simulink model "untitled"  (Simulink 7.5)
settings: Solver=ode45  StartTime=0.0  StopTime=1.4  RelTol=1e-3
libraries: fl_lib x38, nesl_utility x3
settings Model: Creator=USUARIO  LastModifiedBy=davito

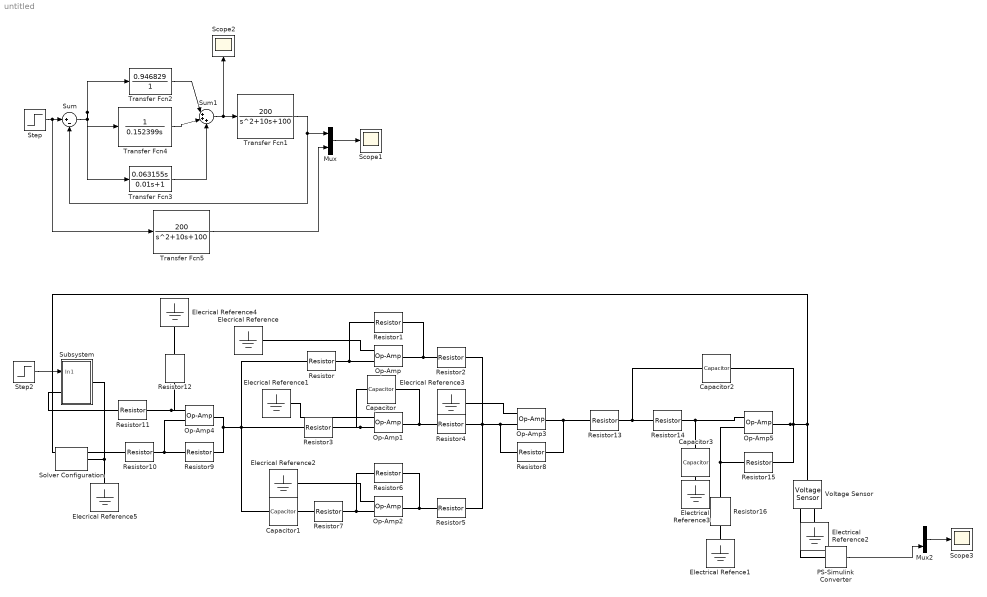
== system untitled ==
  Capacitor : fl_lib/Electrical/Electrical Elements/Capacitor  DialogController=NetworkEngine.DynNeDlgSource  SystemSampleTime=-1  c=10e-6 F  v0=0 V  r=1e-6 Ohm  g=0 1/Ohm  i_Log=off  v_Log=off  vc_Log=off  LocalVarNames=|i|v|vc  LocalVarDescs=|i|v|Internal variable for voltage across capacitor term  LocalVarLogging=[0 0 0]
  Capacitor1 : fl_lib/Electrical/Electrical Elements/Capacitor  DialogController=NetworkEngine.DynNeDlgSource  SystemSampleTime=-1  c=10e-6 F  v0=0 V  r=1e-6 Ohm  g=0 1/Ohm  i_Log=off  v_Log=off  vc_Log=off  LocalVarNames=|i|v|vc  LocalVarDescs=|i|v|Internal variable for voltage across capacitor term  LocalVarLogging=[0 0 0]
  Capacitor2 : fl_lib/Electrical/Electrical Elements/Capacitor  DialogController=NetworkEngine.DynNeDlgSource  SystemSampleTime=-1  c=10.97e-06 F  v0=0 V  r=1e-06 Ohm  g=0 1/Ohm  i_Log=off  v_Log=off  vc_Log=off  LocalVarNames=|i|v|vc  LocalVarDescs=|i|v|Internal variable for voltage across capacitor term  LocalVarLogging=[0 0 0]
  Capacitor3 : fl_lib/Electrical/Electrical Elements/Capacitor  DialogController=NetworkEngine.DynNeDlgSource  SystemSampleTime=-1  c=10.49e-06 F  v0=0 V  r=1e-06 Ohm  g=0 1/Ohm  i_Log=off  v_Log=off  vc_Log=off  LocalVarNames=|i|v|vc  LocalVarDescs=|i|v|Internal variable for voltage across capacitor term  LocalVarLogging=[0 0 0]
  Elecrical Reference{,1..5} (6 alike) : fl_lib/Electrical/Electrical Elements/Electrical Reference  DialogController=NetworkEngine.DynNeDlgSource  SystemSampleTime=-1  i_Log=off  LocalVarNames=|i  LocalVarDescs=|i  LocalVarLogging=0
  Electrical Refence1 : fl_lib/Electrical/Electrical Elements/Electrical Reference  DialogController=NetworkEngine.DynNeDlgSource  SystemSampleTime=-1  i_Log=off  LocalVarNames=|i  LocalVarDescs=|i  LocalVarLogging=0
  Electrical Reference2 : fl_lib/Electrical/Electrical Elements/Electrical Reference  DialogController=NetworkEngine.DynNeDlgSource  SystemSampleTime=-1  i_Log=off  LocalVarNames=|i  LocalVarDescs=|i  LocalVarLogging=0
  Electrical Reference3 : fl_lib/Electrical/Electrical Elements/Electrical Reference  DialogController=NetworkEngine.DynNeDlgSource  SystemSampleTime=-1  i_Log=off  LocalVarNames=|i  LocalVarDescs=|i  LocalVarLogging=0
  Mux : Mux  Inputs=2
  Mux2 : Mux  Inputs=2
  Op-Amp{,1..5} (6 alike) : fl_lib/Electrical/Electrical Elements/Op-Amp  DialogController=NetworkEngine.DynNeDlgSource  SystemSampleTime=-1  i1_Log=off  v1_Log=off  outI_Log=off  LocalVarNames=|i1|v1|outI  LocalVarDescs=|i1|v1|outI  LocalVarLogging=[0 0 0]
  PS-Simulink Converter : nesl_utility/PS-Simulink Converter  DialogController=NetworkEngine.DynNeUtilDlgSource  SystemSampleTime=-1  PhysicalDomain=network_engine_domain  LeftPortType=input  RightPortType=output  SubClassName=ps_output  Unit=1  AffineConversion=off
  Resistor{,2,4..5,7..12} (10 alike) : fl_lib/Electrical/Electrical Elements/Resistor  DialogController=NetworkEngine.DynNeDlgSource  SystemSampleTime=-1  R=1 kOhm  i_Log=off  v_Log=off  LocalVarNames=|i|v  LocalVarDescs=|i|v  LocalVarLogging=[0 0]
  Resistor1 : fl_lib/Electrical/Electrical Elements/Resistor  DialogController=NetworkEngine.DynNeDlgSource  SystemSampleTime=-1  R=946.829 Ohm  i_Log=off  v_Log=off  LocalVarNames=|i|v  LocalVarDescs=|i|v  LocalVarLogging=[0 0]
  Resistor13 : fl_lib/Electrical/Electrical Elements/Resistor  DialogController=NetworkEngine.DynNeDlgSource  SystemSampleTime=-1  R=10.04 kOhm  i_Log=off  v_Log=off  LocalVarNames=|i|v  LocalVarDescs=|i|v  LocalVarLogging=[0 0]
  Resistor14 : fl_lib/Electrical/Electrical Elements/Resistor  DialogController=NetworkEngine.DynNeDlgSource  SystemSampleTime=-1  R=10.03 kOhm  i_Log=off  v_Log=off  LocalVarNames=|i|v  LocalVarDescs=|i|v  LocalVarLogging=[0 0]
  Resistor15 : fl_lib/Electrical/Electrical Elements/Resistor  DialogController=NetworkEngine.DynNeDlgSource  SystemSampleTime=-1  R=4.61 kOhm  i_Log=off  v_Log=off  LocalVarNames=|i|v  LocalVarDescs=|i|v  LocalVarLogging=[0 0]
  Resistor16 : fl_lib/Electrical/Electrical Elements/Resistor  DialogController=NetworkEngine.DynNeDlgSource  SystemSampleTime=-1  R=4.72 kOhm  i_Log=off  v_Log=off  LocalVarNames=|i|v  LocalVarDescs=|i|v  LocalVarLogging=[0 0]
  Resistor3 : fl_lib/Electrical/Electrical Elements/Resistor  DialogController=NetworkEngine.DynNeDlgSource  SystemSampleTime=-1  R=15239.9 Ohm  i_Log=off  v_Log=off  LocalVarNames=|i|v  LocalVarDescs=|i|v  LocalVarLogging=[0 0]
  Resistor6 : fl_lib/Electrical/Electrical Elements/Resistor  DialogController=NetworkEngine.DynNeDlgSource  SystemSampleTime=-1  R=6315.5 Ohm  i_Log=off  v_Log=off  LocalVarNames=|i|v  LocalVarDescs=|i|v  LocalVarLogging=[0 0]
  Scope1 : Scope
  Scope2 : Scope
  Scope3 : Scope
      settings: SaveName=ScopeData2
  Solver Configuration : nesl_utility/Solver Configuration  DialogController=NetworkEngine.DynNeUtilDlgSource  SystemSampleTime=-1  PhysicalDomain=network_engine_domain  LeftPortType=input  RightPortType=generic  SubClassName=solver  Accelerate=off  Profile=off  ResidualTolerance=1e-9  MaxNonlinIter=12  MaxModeIter=2  DoFixedCost=off  UseLocalSampling=off  DoDC=off  LinearAlgebra=Sparse  LocalSolverSampleTime=.001  LocalSolverChoice=NE_BACKWARD_EULER_ADVANCER  UseLocalSolver=off
  Step : Step  Time=0  SampleTime=0
  Step2 : Step  Time=0  SampleTime=0
  Subsystem : Subsystem
  Sum : Sum  Inputs=|+-
  Sum1 : Sum  Inputs=|+++
  Transfer Fcn1 : TransferFcn  Numerator=[200]  Denominator=[1 10 100]
  Transfer Fcn2 : TransferFcn  Numerator=[0.946829]  Denominator=[1]
  Transfer Fcn3 : TransferFcn  Numerator=[0.063155 0]  Denominator=[0.01 1]
  Transfer Fcn4 : TransferFcn  Denominator=[0.152399 0]
  Transfer Fcn5 : TransferFcn  Numerator=[200]  Denominator=[1 10 100]
  Voltage Sensor : fl_lib/Electrical/Electrical Sensors/Voltage Sensor  DialogController=NetworkEngine.DynNeDlgSource  SystemSampleTime=-1  i1_Log=off  v1_Log=off  LocalVarNames=|i1|v1  LocalVarDescs=|i1|v1  LocalVarLogging=[0 0]
  wires:
  Transfer Fcn2/1 -> Sum1/1
  Transfer Fcn4/1 -> Sum1/2
  Transfer Fcn3/1 -> Sum1/3
  Transfer Fcn1/1 -> Sum/2, Mux/1
  Step/1 -> Sum/1, Transfer Fcn5/1
  Sum/1 -> Transfer Fcn2/1, Transfer Fcn4/1, Transfer Fcn3/1
  Sum1/1 -> Transfer Fcn1/1, Scope2/1
  Transfer Fcn5/1 -> Mux/2
  Mux/1 -> Scope1/1
  Step2/1 -> Subsystem/1(In1)
  Mux2/1 -> Scope3/1
  PS-Simulink Converter/1 -> Mux2/2
  connections:
  Op-Amp/LConn2 -- Resistor/RConn1 -- Resistor1/LConn1
  Op-Amp1/LConn2 -- Resistor3/RConn1 -- Capacitor/LConn1
  Op-Amp2/LConn2 -- Resistor7/RConn1 -- Resistor6/LConn1
  Op-Amp2/RConn1 -- Resistor5/LConn1 -- Resistor6/RConn1
  Op-Amp1/RConn1 -- Resistor4/LConn1 -- Capacitor/RConn1
  Op-Amp/RConn1 -- Resistor2/LConn1 -- Resistor1/RConn1
  Capacitor1/RConn1 -- Resistor7/LConn1
  Resistor9/RConn1 -- Capacitor1/LConn1 -- Resistor3/LConn1 -- Resistor/LConn1 -- Op-Amp4/RConn1
  Resistor5/RConn1 -- Resistor4/RConn1 -- Resistor2/RConn1 -- Op-Amp3/LConn2 -- Resistor8/LConn1
  Resistor8/RConn1 -- Op-Amp3/RConn1 -- Resistor13/LConn1
  Elecrical Reference/LConn1 -- Op-Amp/LConn1
  Elecrical Reference2/LConn1 -- Op-Amp2/LConn1
  Elecrical Reference1/LConn1 -- Op-Amp1/LConn1
  Elecrical Reference3/LConn1 -- Op-Amp3/LConn1
  Elecrical Reference4/LConn1 -- Resistor12/RConn1
  Resistor11/RConn1 -- Op-Amp4/LConn1 -- Resistor12/LConn1
  Resistor9/LConn1 -- Resistor10/RConn1 -- Op-Amp4/LConn2
  Capacitor2/LConn1 -- Resistor14/LConn1 -- Resistor13/RConn1
  Op-Amp5/LConn2 -- Resistor16/LConn1 -- Resistor15/LConn1
  Capacitor3/LConn1 -- Resistor14/RConn1 -- Op-Amp5/LConn1
  Resistor15/RConn1 -- Capacitor2/RConn1 -- Op-Amp5/RConn1 -- Voltage Sensor/LConn1 -- Resistor10/LConn1
  Electrical Reference3/LConn1 -- Capacitor3/RConn1
  Electrical Refence1/LConn1 -- Resistor16/RConn1
  Voltage Sensor/RConn2 -- Electrical Reference2/LConn1
  Voltage Sensor/RConn1 -- PS-Simulink Converter/LConn1
  Subsystem/RConn1 -- Elecrical Reference5/LConn1 -- Solver Configuration/RConn1
  Subsystem/LConn1 -- Resistor11/LConn1

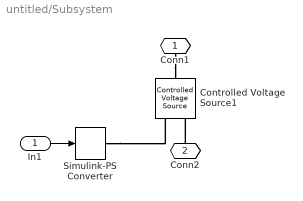
== system untitled/Subsystem ==
  In1 : Inport
  Controlled Voltage Source1 : fl_lib/Electrical/Electrical Sources/Controlled Voltage Source  DialogController=NetworkEngine.DynNeDlgSource  SystemSampleTime=-1  i_Log=off  v_Log=off  LocalVarNames=|i|v  LocalVarDescs=|i|v  LocalVarLogging=[0 0]
  Simulink-PS Converter : nesl_utility/Simulink-PS Converter  DialogController=NetworkEngine.DynNeUtilDlgSource  SystemSampleTime=-1  PhysicalDomain=network_engine_domain  LeftPortType=input  RightPortType=output  SubClassName=ps_input  Unit=1  AffineConversion=off  InputFilterTimeConstant=.001  UdotUserProvided=0
  Conn1 : PMIOPort  Port=1  Side=Left
  Conn2 : PMIOPort  Port=2  Side=Right
  wires:
  In1/1 -> Simulink-PS Converter/1
  connections:
  Simulink-PS Converter/RConn1 -- Controlled Voltage Source1/RConn1
  Conn1/RConn1 -- Controlled Voltage Source1/LConn1
  Conn2/RConn1 -- Controlled Voltage Source1/RConn2
